simulink model "matlab_forward_back_Correcting_moni"  (R2018b)
settings: Solver=VariableStepAuto  StartTime=0.0  StopTime=80  RelTol=1e-3
settings Model: Creator=erange  LastModifiedBy=erange

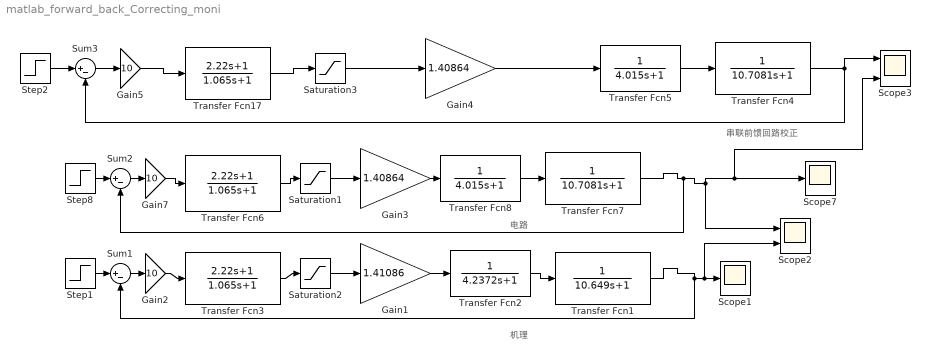
== system matlab_forward_back_Correcting_moni ==
  note: 机理
  note: 电路
  note: 串联前馈回路校正
  Gain1 : Gain  Gain=1.41086
  Gain2 : Gain  Gain=10
  Gain3 : Gain  Gain=1.40864
  Gain4 : Gain  Gain=1.40864
  Gain5 : Gain  Gain=10
  Gain7 : Gain  Gain=10
  Saturation1 : Saturate  UpperLimit=5  LowerLimit=0
  Saturation2 : Saturate  UpperLimit=5  LowerLimit=0
  Saturation3 : Saturate  UpperLimit=5  LowerLimit=0
  Scope1 : Scope
  Scope2 : Scope  NumInputPorts=2
  Scope3 : Scope  NumInputPorts=2
  Scope7 : Scope
  Step1 : Step  Time=0  SampleTime=0
  Step2 : Step  Time=0  SampleTime=0
  Step8 : Step  Time=0  SampleTime=0
  Sum1 : Sum  Inputs=|+-
  Sum2 : Sum  Inputs=|+-
  Sum3 : Sum  Inputs=|+-
  Transfer Fcn1 : TransferFcn  Denominator=[10.649 1]
  Transfer Fcn17 : TransferFcn  Numerator=[2.22 1]  Denominator=[1.065 1]
  Transfer Fcn2 : TransferFcn  Denominator=[4.2372 1]
  Transfer Fcn3 : TransferFcn  Numerator=[2.22 1]  Denominator=[1.065 1]
  Transfer Fcn4 : TransferFcn  Denominator=[10.7081 1]
  Transfer Fcn5 : TransferFcn  Denominator=[4.015 1]
  Transfer Fcn6 : TransferFcn  Numerator=[2.22 1]  Denominator=[1.065 1]
  Transfer Fcn7 : TransferFcn  Denominator=[10.7081 1]
  Transfer Fcn8 : TransferFcn  Denominator=[4.015 1]
  wires:
  Sum2/1 -> Gain7/1
  Saturation1/1 -> Gain3/1
  Step8/1 -> Sum2/1
  Transfer Fcn1/1 -> Sum1/2, Scope2/2, Scope1/1
  Transfer Fcn3/1 -> Saturation2/1
  Gain1/1 -> Transfer Fcn2/1
  Saturation2/1 -> Gain1/1
  Gain2/1 -> Transfer Fcn3/1
  Step1/1 -> Sum1/1
  Transfer Fcn2/1 -> Transfer Fcn1/1
  Sum1/1 -> Gain2/1
  Gain3/1 -> Transfer Fcn8/1
  Transfer Fcn8/1 -> Transfer Fcn7/1
  Transfer Fcn7/1 -> Sum2/2, Scope2/1, Scope3/2, Scope7/1
  Gain4/1 -> Transfer Fcn5/1
  Step2/1 -> Sum3/1
  Sum3/1 -> Gain5/1
  Saturation3/1 -> Gain4/1
  Transfer Fcn5/1 -> Transfer Fcn4/1
  Transfer Fcn4/1 -> Scope3/1, Sum3/2
  Gain5/1 -> Transfer Fcn17/1
  Transfer Fcn17/1 -> Saturation3/1
  Gain7/1 -> Transfer Fcn6/1
  Transfer Fcn6/1 -> Saturation1/1
